simulink model "Speed_Quintic_Controller"  (R2021a)
settings: Solver=VariableStepAuto  StartTime=0.0  StopTime=0.7  MaxStep=.01  RelTol=1e-3  AbsTol=1e-3
undefined symbols (not defined in the file): a_ret, Angle_noise, Current_noise, efficiency, F_sampling, J_load, J_rotor, km, n, q_ret, smiData, T_fin, T_ramp, T_ret, Velocity_noise, W_cruise, X, Y, Z
libraries: sm_lib x99, nesl_utility x12, fl_lib x11, simulink x3, spsSampleandHoldLib x3, ee_lib x3, pid_lib x3, sdl_lib x1
(part 3 of 3)

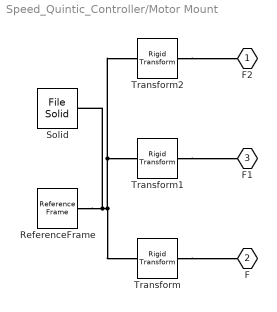
== system Speed_Quintic_Controller/Motor Mount ==
  ReferenceFrame : sm_lib/Frames and Transforms/Reference Frame
  Solid : sm_lib/Body Elements/File Solid  ExtGeomFileName=8982K141_Multipurpose 6061 Aluminum 90 Degree Angle_8982K141_sldprt.STEP  UnitType=FromFile  ExtGeomFileUnits=m  StepReaderType=HEX  ExportConvexHullGeometry=off  InertiaType=Custom  Mass=smiData.Solid(7).mass  MassUnits=kg  CenterOfMass=smiData.Solid(7).CoM  CenterOfMassUnits=in  MomentsOfInertia=smiData.Solid(7).MoI  MomentsOfInertiaUnits=kg*in^2  ProductsOfInertia=smiData.Solid(7).PoI  ProductsOfInertiaUnits=kg*in^2  BasedOnType=DensityFromFile  Density=1000  DensityUnits=kg/m^3  DoExposeReferenceFrame=on  SerializedFrames=<Frames/>  GraphicType=FromGeometry  MarkerShape=Sphere  MarkerSize=10  GraphicVisPropType=SimpleVisualProperties  GraphicDiffuseColor=smiData.Solid(7).color  GraphicSpecularColor=[0.5 0.5 0.5 1.0]  GraphicAmbientColor=[0.15 0.15 0.15 1.0]  GraphicEmissiveColor=[0.0 0.0 0.0 1.0]  GraphicShininess=75  GraphicOpacity=smiData.Solid(7).opacity
  Transform : sm_lib/Frames and Transforms/Rigid Transform  TranslationMethod=Cartesian  TranslationStandardOffset=0  TranslationLengthUnit=mm  TranslationStandardAxis=+Z  TranslationCartesianOffset=smiData.RigidTransform(24).translation  TranslationROffset=0  TranslationROffsetUnits=m  TranslationZOffset=0  TranslationZOffsetUnits=m  TranslationThetaOffset=0  TranslationThetaOffsetUnits=deg  RotationMethod=ArbitraryAxis  RotationAngleUnits=rad  RotationStandardAxis=+Z  RotationAngle=smiData.RigidTransform(24).angle  RotationArbitraryAxis=smiData.RigidTransform(24).axis  FollAlignAxisA=+X  BaseAlignAxisA=+Y  FollAlignAxisB=+Y  BaseAlignAxisB=+Z  RotationSequenceAxes=FollowerAxes  RotationSequence=XYX  RotationSequenceAngles=[0 0 0]  RotationSequenceAnglesUnits=deg  RotationMatrix=[1 0 0; 0 1 0; 0 0 1]
  Transform1 : sm_lib/Frames and Transforms/Rigid Transform  TranslationMethod=Cartesian  TranslationStandardOffset=0  TranslationLengthUnit=mm  TranslationStandardAxis=+Z  TranslationCartesianOffset=smiData.RigidTransform(25).translation  TranslationROffset=0  TranslationROffsetUnits=m  TranslationZOffset=0  TranslationZOffsetUnits=m  TranslationThetaOffset=0  TranslationThetaOffsetUnits=deg  RotationMethod=ArbitraryAxis  RotationAngleUnits=rad  RotationStandardAxis=+Z  RotationAngle=smiData.RigidTransform(25).angle  RotationArbitraryAxis=smiData.RigidTransform(25).axis  FollAlignAxisA=+X  BaseAlignAxisA=+Y  FollAlignAxisB=+Y  BaseAlignAxisB=+Z  RotationSequenceAxes=FollowerAxes  RotationSequence=XYX  RotationSequenceAngles=[0 0 0]  RotationSequenceAnglesUnits=deg  RotationMatrix=[1 0 0; 0 1 0; 0 0 1]
  Transform2 : sm_lib/Frames and Transforms/Rigid Transform  TranslationMethod=Cartesian  TranslationStandardOffset=0  TranslationLengthUnit=mm  TranslationStandardAxis=+Z  TranslationCartesianOffset=smiData.RigidTransform(42).translation  TranslationROffset=0  TranslationROffsetUnits=m  TranslationZOffset=0  TranslationZOffsetUnits=m  TranslationThetaOffset=0  TranslationThetaOffsetUnits=deg  RotationMethod=ArbitraryAxis  RotationAngleUnits=rad  RotationStandardAxis=+Z  RotationAngle=smiData.RigidTransform(42).angle  RotationArbitraryAxis=smiData.RigidTransform(42).axis  FollAlignAxisA=+X  BaseAlignAxisA=+Y  FollAlignAxisB=+Y  BaseAlignAxisB=+Z  RotationSequenceAxes=FollowerAxes  RotationSequence=XYX  RotationSequenceAngles=[0 0 0]  RotationSequenceAnglesUnits=deg  RotationMatrix=[1 0 0; 0 1 0; 0 0 1]
  F2 : PMIOPort  Side=Left
  F : PMIOPort  Port=2  Side=Left
  F1 : PMIOPort  Port=3  Side=Right
  connections:
  Solid/RConn1 -- ReferenceFrame/RConn1 -- Transform1/LConn1 -- Transform2/LConn1 -- Transform/LConn1
  Transform/RConn1 -- F/RConn1
  Transform1/RConn1 -- F1/RConn1
  Transform2/RConn1 -- F2/RConn1

== system Speed_Quintic_Controller/Output Gear ==
  ReferenceFrame : sm_lib/Frames and Transforms/Reference Frame
  Solid : sm_lib/Body Elements/File Solid  ExtGeomFileName=2664N150_METAL GEAR - 20 DEGREE PRESSURE ANGLE_2664N15_sldprt.STEP  UnitType=FromFile  ExtGeomFileUnits=m  StepReaderType=HEX  ExportConvexHullGeometry=off  InertiaType=Custom  Mass=smiData.Solid(3).mass  MassUnits=kg  CenterOfMass=smiData.Solid(3).CoM  CenterOfMassUnits=in  MomentsOfInertia=smiData.Solid(3).MoI  MomentsOfInertiaUnits=kg*in^2  ProductsOfInertia=smiData.Solid(3).PoI  ProductsOfInertiaUnits=kg*in^2  BasedOnType=DensityFromFile  Density=1000  DensityUnits=kg/m^3  DoExposeReferenceFrame=on  SerializedFrames=<Frames/>  GraphicType=FromGeometry  MarkerShape=Sphere  MarkerSize=10  GraphicVisPropType=SimpleVisualProperties  GraphicDiffuseColor=smiData.Solid(3).color  GraphicSpecularColor=[0.5 0.5 0.5 1.0]  GraphicAmbientColor=[0.15 0.15 0.15 1.0]  GraphicEmissiveColor=[0.0 0.0 0.0 1.0]  GraphicShininess=75  GraphicOpacity=smiData.Solid(3).opacity
  Transform : sm_lib/Frames and Transforms/Rigid Transform  TranslationMethod=Cartesian  TranslationStandardOffset=0  TranslationLengthUnit=mm  TranslationStandardAxis=+Z  TranslationCartesianOffset=smiData.RigidTransform(38).translation  TranslationROffset=0  TranslationROffsetUnits=m  TranslationZOffset=0  TranslationZOffsetUnits=m  TranslationThetaOffset=0  TranslationThetaOffsetUnits=deg  RotationMethod=ArbitraryAxis  RotationAngleUnits=rad  RotationStandardAxis=+Z  RotationAngle=smiData.RigidTransform(38).angle  RotationArbitraryAxis=smiData.RigidTransform(38).axis  FollAlignAxisA=+X  BaseAlignAxisA=+Y  FollAlignAxisB=+Y  BaseAlignAxisB=+Z  RotationSequenceAxes=FollowerAxes  RotationSequence=XYX  RotationSequenceAngles=[0 0 0]  RotationSequenceAnglesUnits=deg  RotationMatrix=[1 0 0; 0 1 0; 0 0 1]
  Transform1 : sm_lib/Frames and Transforms/Rigid Transform  TranslationMethod=Cartesian  TranslationStandardOffset=0  TranslationLengthUnit=mm  TranslationStandardAxis=+Z  TranslationCartesianOffset=smiData.RigidTransform(39).translation  TranslationROffset=0  TranslationROffsetUnits=m  TranslationZOffset=0  TranslationZOffsetUnits=m  TranslationThetaOffset=0  TranslationThetaOffsetUnits=deg  RotationMethod=ArbitraryAxis  RotationAngleUnits=rad  RotationStandardAxis=+Z  RotationAngle=smiData.RigidTransform(39).angle  RotationArbitraryAxis=smiData.RigidTransform(39).axis  FollAlignAxisA=+X  BaseAlignAxisA=+Y  FollAlignAxisB=+Y  BaseAlignAxisB=+Z  RotationSequenceAxes=FollowerAxes  RotationSequence=XYX  RotationSequenceAngles=[0 0 0]  RotationSequenceAnglesUnits=deg  RotationMatrix=[1 0 0; 0 1 0; 0 0 1]
  F : PMIOPort  Side=Left
  F1 : PMIOPort  Port=2  Side=Left
  connections:
  Solid/RConn1 -- ReferenceFrame/RConn1 -- Transform/LConn1 -- Transform1/LConn1
  Transform/RConn1 -- F/RConn1
  Transform1/RConn1 -- F1/RConn1

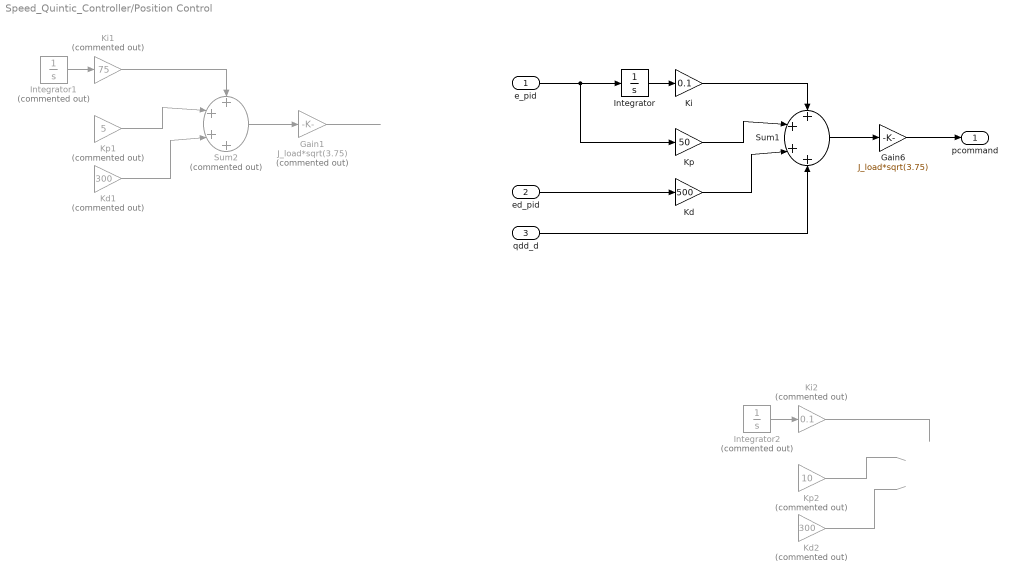
== system Speed_Quintic_Controller/Position Control ==
  e_pid : Inport
  ed_pid : Inport  Port=2
  qdd_d : Inport  Port=3
  Gain1 : Gain  Commented=on  Gain=J_load*sqrt(3.75)
  Gain6 : Gain  Gain=J_load*sqrt(3.75)
  Integrator : Integrator
  Integrator1 : Integrator  Commented=on
  Integrator2 : Integrator  Commented=on
  Kd : Gain  Gain=500
  Kd1 : Gain  Commented=on  Gain=300
  Kd2 : Gain  Commented=on  Gain=300
  Ki : Gain  Gain=0.1
  Ki1 : Gain  Commented=on  Gain=75
  Ki2 : Gain  Commented=on  Gain=0.1
  Kp : Gain  Gain=50
  Kp1 : Gain  Commented=on  Gain=5
  Kp2 : Gain  Commented=on  Gain=10
  Sum1 : Sum  Inputs=++++
  Sum2 : Sum  Commented=on  Inputs=++++
  pcommand : Outport
  wires:
  e_pid/1 -> Integrator/1, Kp/1
  qdd_d/1 -> Sum1/4
  ed_pid/1 -> Kd/1
  Integrator/1 -> Ki/1
  Sum1/1 -> Gain6/1
  Kp/1 -> Sum1/2
  Gain6/1 -> pcommand/1
  Ki/1 -> Sum1/1
  Kd/1 -> Sum1/3
  Kp1/1 -> Sum2/2
  Ki1/1 -> Sum2/1
  Sum2/1 -> Gain1/1
  Kd1/1 -> Sum2/3
  ? -> Integrator1/1, Kp1/1
  ? -> Kd1/1
  Integrator1/1 -> Ki1/1
  ? -> Sum2/4
  Gain1/1 -> ?
  ? -> Kd2/1
  ? -> Integrator2/1, Kp2/1
  Kd2/1 -> ?
  Ki2/1 -> ?
  Integrator2/1 -> Ki2/1
  Kp2/1 -> ?
  ? -> ?

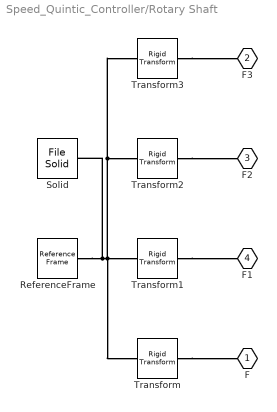
== system Speed_Quintic_Controller/Rotary Shaft ==
  ReferenceFrame : sm_lib/Frames and Transforms/Reference Frame
  Solid : sm_lib/Body Elements/File Solid  ExtGeomFileName=1439K411_1045 Carbon Steel Keyed Rotary Shaft_1439K411_sldprt.STEP  UnitType=FromFile  ExtGeomFileUnits=m  StepReaderType=HEX  ExportConvexHullGeometry=off  InertiaType=Custom  Mass=smiData.Solid(9).mass  MassUnits=kg  CenterOfMass=smiData.Solid(9).CoM  CenterOfMassUnits=mm  MomentsOfInertia=smiData.Solid(9).MoI  MomentsOfInertiaUnits=kg*mm^2  ProductsOfInertia=smiData.Solid(9).PoI  ProductsOfInertiaUnits=kg*mm^2  BasedOnType=DensityFromFile  Density=1000  DensityUnits=kg/m^3  DoExposeReferenceFrame=on  SerializedFrames=<Frames/>  GraphicType=FromGeometry  MarkerShape=Sphere  MarkerSize=10  GraphicVisPropType=SimpleVisualProperties  GraphicDiffuseColor=smiData.Solid(9).color  GraphicSpecularColor=[0.5 0.5 0.5 1.0]  GraphicAmbientColor=[0.15 0.15 0.15 1.0]  GraphicEmissiveColor=[0.0 0.0 0.0 1.0]  GraphicShininess=75  GraphicOpacity=smiData.Solid(9).opacity
  Transform : sm_lib/Frames and Transforms/Rigid Transform  TranslationMethod=Cartesian  TranslationStandardOffset=0  TranslationLengthUnit=mm  TranslationStandardAxis=+Z  TranslationCartesianOffset=smiData.RigidTransform(22).translation  TranslationROffset=0  TranslationROffsetUnits=m  TranslationZOffset=0  TranslationZOffsetUnits=m  TranslationThetaOffset=0  TranslationThetaOffsetUnits=deg  RotationMethod=ArbitraryAxis  RotationAngleUnits=rad  RotationStandardAxis=+Z  RotationAngle=smiData.RigidTransform(22).angle  RotationArbitraryAxis=smiData.RigidTransform(22).axis  FollAlignAxisA=+X  BaseAlignAxisA=+Y  FollAlignAxisB=+Y  BaseAlignAxisB=+Z  RotationSequenceAxes=FollowerAxes  RotationSequence=XYX  RotationSequenceAngles=[0 0 0]  RotationSequenceAnglesUnits=deg  RotationMatrix=[1 0 0; 0 1 0; 0 0 1]
  Transform1 : sm_lib/Frames and Transforms/Rigid Transform  TranslationMethod=Cartesian  TranslationStandardOffset=0  TranslationLengthUnit=mm  TranslationStandardAxis=+Z  TranslationCartesianOffset=smiData.RigidTransform(27).translation  TranslationROffset=0  TranslationROffsetUnits=m  TranslationZOffset=0  TranslationZOffsetUnits=m  TranslationThetaOffset=0  TranslationThetaOffsetUnits=deg  RotationMethod=ArbitraryAxis  RotationAngleUnits=rad  RotationStandardAxis=+Z  RotationAngle=smiData.RigidTransform(27).angle  RotationArbitraryAxis=smiData.RigidTransform(27).axis  FollAlignAxisA=+X  BaseAlignAxisA=+Y  FollAlignAxisB=+Y  BaseAlignAxisB=+Z  RotationSequenceAxes=FollowerAxes  RotationSequence=XYX  RotationSequenceAngles=[0 0 0]  RotationSequenceAnglesUnits=deg  RotationMatrix=[1 0 0; 0 1 0; 0 0 1]
  Transform2 : sm_lib/Frames and Transforms/Rigid Transform  TranslationMethod=Cartesian  TranslationStandardOffset=0  TranslationLengthUnit=mm  TranslationStandardAxis=+Z  TranslationCartesianOffset=smiData.RigidTransform(35).translation  TranslationROffset=0  TranslationROffsetUnits=m  TranslationZOffset=0  TranslationZOffsetUnits=m  TranslationThetaOffset=0  TranslationThetaOffsetUnits=deg  RotationMethod=ArbitraryAxis  RotationAngleUnits=rad  RotationStandardAxis=+Z  RotationAngle=smiData.RigidTransform(35).angle  RotationArbitraryAxis=smiData.RigidTransform(35).axis  FollAlignAxisA=+X  BaseAlignAxisA=+Y  FollAlignAxisB=+Y  BaseAlignAxisB=+Z  RotationSequenceAxes=FollowerAxes  RotationSequence=XYX  RotationSequenceAngles=[0 0 0]  RotationSequenceAnglesUnits=deg  RotationMatrix=[1 0 0; 0 1 0; 0 0 1]
  Transform3 : sm_lib/Frames and Transforms/Rigid Transform  TranslationMethod=Cartesian  TranslationStandardOffset=0  TranslationLengthUnit=mm  TranslationStandardAxis=+Z  TranslationCartesianOffset=smiData.RigidTransform(37).translation  TranslationROffset=0  TranslationROffsetUnits=m  TranslationZOffset=0  TranslationZOffsetUnits=m  TranslationThetaOffset=0  TranslationThetaOffsetUnits=deg  RotationMethod=ArbitraryAxis  RotationAngleUnits=rad  RotationStandardAxis=+Z  RotationAngle=smiData.RigidTransform(37).angle  RotationArbitraryAxis=smiData.RigidTransform(37).axis  FollAlignAxisA=+X  BaseAlignAxisA=+Y  FollAlignAxisB=+Y  BaseAlignAxisB=+Z  RotationSequenceAxes=FollowerAxes  RotationSequence=XYX  RotationSequenceAngles=[0 0 0]  RotationSequenceAnglesUnits=deg  RotationMatrix=[1 0 0; 0 1 0; 0 0 1]
  F : PMIOPort  Side=Left
  F3 : PMIOPort  Port=2  Side=Right
  F2 : PMIOPort  Port=3  Side=Right
  F1 : PMIOPort  Port=4  Side=Right
  connections:
  Solid/RConn1 -- ReferenceFrame/RConn1 -- Transform2/LConn1 -- Transform3/LConn1 -- Transform/LConn1 -- Transform1/LConn1
  Transform/RConn1 -- F/RConn1
  Transform1/RConn1 -- F1/RConn1
  Transform2/RConn1 -- F2/RConn1
  Transform3/RConn1 -- F3/RConn1

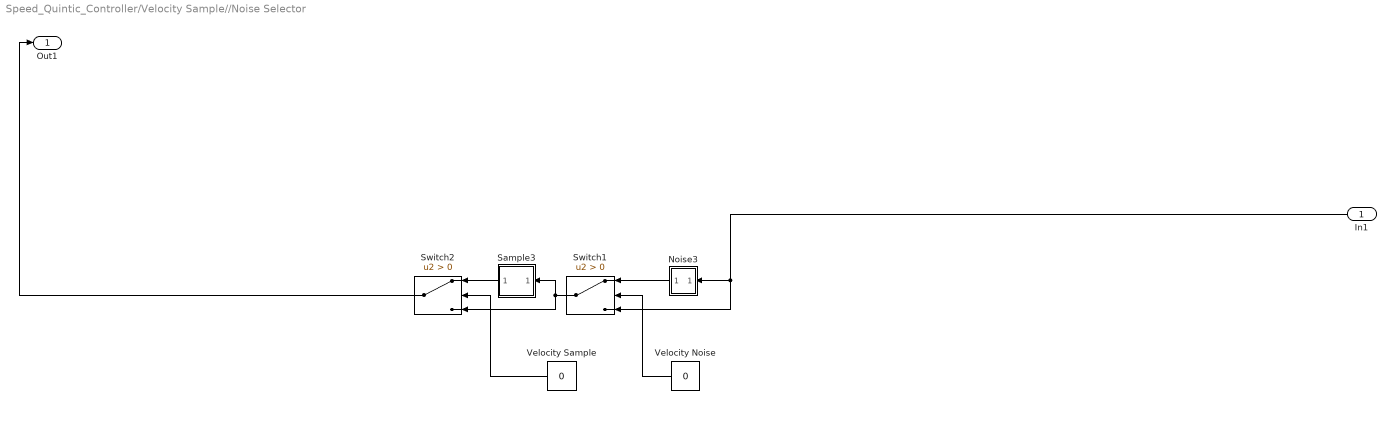
== system Speed_Quintic_Controller/Velocity Sample//Noise Selector ==
  In1 : Inport
  Noise3 : Subsystem
  Sample3 : Subsystem
  Switch1 : Switch  Criteria=u2 > Threshold
  Switch2 : Switch  Criteria=u2 > Threshold
  Velocity Noise : Constant  Value=0
  Velocity Sample : Constant  Value=0
  Out1 : Outport
  wires:
  Switch1/1 -> Switch2/3, Sample3/1(In1)
  Sample3/1("   ") -> Switch2/1
  Velocity Noise/1 -> Switch1/2
  Switch2/1 -> Out1/1
  In1/1 -> Noise3/1(In1), Switch1/3
  Noise3/1(Out1) -> Switch1/1
  Velocity Sample/1 -> Switch2/2

== system Speed_Quintic_Controller/Angle Sample//Noise Selector1/Noise3 ==
  In1 : Inport
  Band-Limited White Noise : simulink/Sources/Band-Limited White Noise  Cov=[Angle_noise]  Ts=0.001  seed=[23341]
  Sum3 : Sum  Inputs=|++
  Out1 : Outport
  wires:
  Band-Limited White Noise/1 -> Sum3/1
  In1/1 -> Sum3/2
  Sum3/1 -> Out1/1

== system Speed_Quintic_Controller/Angle Sample//Noise Selector1/Sample3 ==
  In1 : Inport
  Pulse Generator : DiscretePulseGenerator  PulseType=Time based  Period=1/F_sampling
  Sample and Hold : spsSampleandHoldLib/Sample and Hold  ic=0  Ts=0
      settings: SourceProductBaseCode=PS
  "   " : Outport
  wires:
  Pulse Generator/1 -> Sample and Hold/2
  Sample and Hold/1 -> "   "/1
  In1/1 -> Sample and Hold/1

== system Speed_Quintic_Controller/Current Sample//Noise Selector/Noise3 ==
  In1 : Inport
  Band-Limited White Noise : simulink/Sources/Band-Limited White Noise  Cov=[Current_noise]  Ts=0.001  seed=[23341]
  Sum3 : Sum  Inputs=|++
  Out1 : Outport
  wires:
  Band-Limited White Noise/1 -> Sum3/1
  In1/1 -> Sum3/2
  Sum3/1 -> Out1/1

== system Speed_Quintic_Controller/Current Sample//Noise Selector/Sample3 ==
  In1 : Inport
  Pulse Generator : DiscretePulseGenerator  PulseType=Time based  Period=1/F_sampling
  Sample and Hold : spsSampleandHoldLib/Sample and Hold  ic=0  Ts=0
      settings: SourceProductBaseCode=PS
  "   " : Outport
  wires:
  Pulse Generator/1 -> Sample and Hold/2
  Sample and Hold/1 -> "   "/1
  In1/1 -> Sample and Hold/1

== system Speed_Quintic_Controller/Velocity Sample//Noise Selector/Noise3 ==
  In1 : Inport
  Band-Limited White Noise : simulink/Sources/Band-Limited White Noise  Cov=[Velocity_noise]  Ts=0.001  seed=[23341]
  Sum3 : Sum  Inputs=|++
  Out1 : Outport
  wires:
  Band-Limited White Noise/1 -> Sum3/1
  In1/1 -> Sum3/2
  Sum3/1 -> Out1/1

== system Speed_Quintic_Controller/Velocity Sample//Noise Selector/Sample3 ==
  In1 : Inport
  Pulse Generator : DiscretePulseGenerator  PulseType=Time based  Period=1/F_sampling
  Sample and Hold : spsSampleandHoldLib/Sample and Hold  ic=0  Ts=0
      settings: SourceProductBaseCode=PS
  "   " : Outport
  wires:
  Pulse Generator/1 -> Sample and Hold/2
  Sample and Hold/1 -> "   "/1
  In1/1 -> Sample and Hold/1

== matlab function Speed_Quintic_Controller/MATLAB Function ==
  data: command input; tau output; pcommand input; theta input; t input; T_ramp input; W_cruise input; T_fin input; T_ret input; a_ret input; q_ret input; omega input; e_pid output; ed_pid output; q_d output; qd_d output; qdd_d output
 function [tau, e_pid, ed_pid, q_d, qd_d, qdd_d] = fcn(command, pcommand, theta, t, T_ramp, W_cruise, T_fin, T_ret, a_ret, q_ret, omega)
 
 if (t <= T_ramp)
     q_d = 0.5 * W_cruise * t^2/T_ramp;
     qd_d = W_cruise * t/T_ramp;
     qdd_d = W_cruise/T_ramp;
     e_pid = qd_d - omega;
     tau = command;
     q_0=[];
     q_1=[];
     q_2=[];
     q_3=[];
     ed_pid = 0;
     
 elseif (t > T_ramp & t < T_ret)
     q_d = 0.5 * W_cruise * T_ramp + W_cruise * (t-T_ramp);
     qd_d = W_cruise;
     qdd_d = 0;
     e_pid = qd_d - omega;
     tau = command;
     q_0=[];
     q_1=[];
     q_2=[];
     q_3=[];
     ed_pid = 0;
     
 elseif (t >= T_ret & t < T_fin)
     Del = T_fin - T_ret;
     q_2 = a_ret*0.5;
     q_1 = W_cruise;
     q_0 = q_ret;
     ii = inv([Del^3 Del^4 Del^5; 3*Del^2 4*Del^3 5*Del^4; 6*Del 12*Del^2 20*Del^3])*[(-q_0 - q_1*Del - q_2*Del^2); (-q_1 - 2*q_2*Del); -2*q_2];
     
     q_3=ii(1); q_4=ii(2); q_5=ii(3);
     Del_T= t- T_ret;
     
     q_d = q_0 + q_1*Del_T + q_2*Del_T^2 + q_3*Del_T^3 + q_4*Del_T^4 + q_5*Del_T^5;
     qd_d = q_1 + 2*q_2*Del_T + 3*q_3*Del_T^2 + 4*q_4*Del_T^3 + 5*q_5*Del_T^4;
     qdd_d = 2*q_2 + 6*q_3*Del_T + 12*q_4*Del_T^2 + 20*q_5*Del_T^3;
     e_pid = q_d - theta;
     ed_pid = qd_d - omega;
     tau = pcommand;
    
 else 
     q_d = 0;
     qd_d = 0;
     qdd_d = 0;
     e_pid = q_d - theta;
     ed_pid = qd_d - omega;
     tau = pcommand;
 end
